simulink model "speed_km_per_hr_to_rpm"  (R2020b)
settings: Solver=VariableStepAuto  StartTime=0.0  StopTime=10.0  RelTol=1e-3
settings Model: Creator=Training  LastModifiedBy=Training

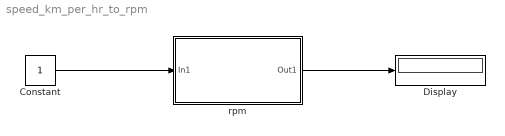
== system speed_km_per_hr_to_rpm ==
  Constant : Constant
  Display : Display
  rpm : Subsystem
  wires:
  rpm/1(Out1) -> Display/1
  Constant/1 -> rpm/1(In1)

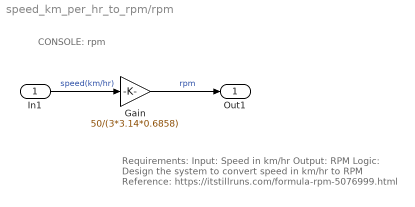
== system speed_km_per_hr_to_rpm/rpm ==
  note: CONSOLE: rpm
  note: Requirements:
      | Input: Speed in km/hr
      | Output: RPM
      | Logic: Design the system to convert speed in km/hr to RPM Reference: https://itstillruns.com/formula-rpm-5076999.html
  In1 : Inport
  Gain : Gain  Gain=50/(3*3.14*0.6858)
  Out1 : Outport
  wires:
  In1/1 -> Gain/1  "speed(km/hr)"
  Gain/1 -> Out1/1  "rpm"
